simulink model "ILC_controller"  (R2018a)
settings: Solver=VariableStepAuto  StartTime=0.0  StopTime=100  RelTol=1e-3  EnableMultiTasking=on
libraries: simulink x2
settings Model: Creator=HUY  LastModifiedBy=thanhdo
settings OptimizationCC: LifeSpan=inf
settings DebuggingCC: SFUnexpectedBacktrackingDiag=warning  SFNoUnconditionalDefaultTransitionDiag=warning
settings CodeAppCC: StateflowObjectComments=on
settings GRTTargetCC: TargetLangStandard=C89/C90 (ANSI)
settings ConfigComp: CovMetricSettings=dw  CovSaveCumulativeToWorkspaceVar=on  CovSaveSingleToWorkspaceVar=on  CovExternalEMLEnable=off
settings SimscapeCC: SimscapeNormalizeSystem=off

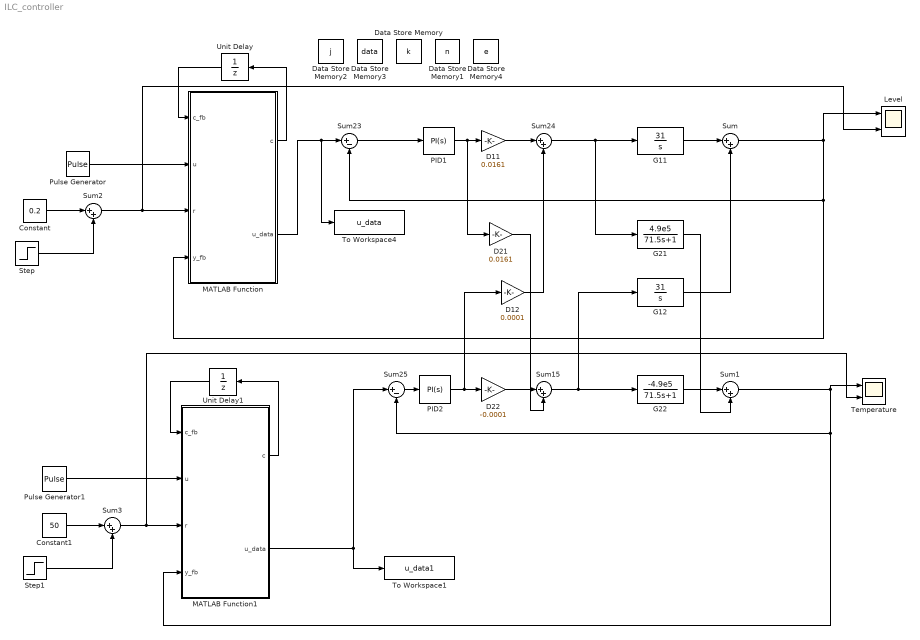
== system ILC_controller ==
  Constant : Constant  Value=0.2
  Constant1 : Constant  Value=50
  D11 : Gain  Gain=0.0161
  D12 : Gain  Gain=0.0001
  D21 : Gain  Gain=0.0161
  D22 : Gain  Gain=-0.0001
  Data Store Memory : DataStoreMemory  DataStoreName=k  ReadBeforeWriteMsg=warning  WriteAfterWriteMsg=warning  WriteAfterReadMsg=warning  ShowAdditionalParam=off  OutDataTypeStr=double
  Data Store Memory1 : DataStoreMemory  DataStoreName=n  ReadBeforeWriteMsg=warning  WriteAfterWriteMsg=warning  WriteAfterReadMsg=warning  ShowAdditionalParam=off  OutDataTypeStr=double
  Data Store Memory2 : DataStoreMemory  DataStoreName=j  ReadBeforeWriteMsg=warning  WriteAfterWriteMsg=warning  WriteAfterReadMsg=warning  ShowAdditionalParam=off  OutDataTypeStr=double
  Data Store Memory3 : DataStoreMemory  DataStoreName=data  ReadBeforeWriteMsg=warning  WriteAfterWriteMsg=warning  WriteAfterReadMsg=warning  ShowAdditionalParam=off  OutDataTypeStr=double  Dimensions=[1 120]
  Data Store Memory4 : DataStoreMemory  DataStoreName=e  ReadBeforeWriteMsg=warning  WriteAfterWriteMsg=warning  WriteAfterReadMsg=warning  ShowAdditionalParam=off  OutDataTypeStr=double  Dimensions=[1 120]
  G11 : TransferFcn  Numerator=[31]  Denominator=[1 0]
  "G12 " : TransferFcn  Numerator=[31]  Denominator=[1 0]
  G21 : TransferFcn  Numerator=[4.9e5]  Denominator=[71.5 1]
  G22 : TransferFcn  Numerator=[-4.9e5]  Denominator=[71.5 1]
  Level : Scope  NumInputPorts=2
  MATLAB Function : MATLAB Function  TreatAsAtomicUnit=on
  MATLAB Function1 : MATLAB Function  TreatAsAtomicUnit=on
  PID1 : simulink/Continuous/PID Controller  Controller=PI  TimeDomain=Continuous-time  SampleTime=-1  IntegratorMethod=Forward Euler  FilterMethod=Forward Euler  Form=Parallel  UseFilter=on  ControllerParametersSource=internal  P=3  I=0.1  D=0  N=100  InitialConditionSource=internal  InitialConditionForIntegrator=0  InitialConditionForFilter=0  ExternalReset=none  LimitOutput=off  UpperSaturationLimit=inf  LowerSaturationLimit=-inf  LinearizeAsGain=on  AntiWindupMode=none  Kb=1  TrackingMode=off  Kt=1  PParamMin=[]  PParamMax=[]  IParamMin=[]  IParamMax=[]  DParamMin=[]  DParamMax=[]  NParamMin=[]  NParamMax=[]  KbParamMin=[]  KbParamMax=[]  KtParamMin=[]  KtParamMax=[]  POutMin=[]  POutMax=[]  IOutMin=[]  IOutMax=[]  DOutMin=[]  DOutMax=[]  NOutMin=[]  NOutMax=[]  KbOutMin=[]  KbOutMax=[]  KtOutMin=[]  KtOutMax=[]  IntegratorOutMin=[]  IntegratorOutMax=[]  FilterOutMin=[]  FilterOutMax=[]  SumOutMin=[]  SumOutMax=[]  SumI1OutMin=[]  SumI1OutMax=[]  SumI2OutMin=[]  SumI2OutMax=[]  SumI3OutMin=[]  SumI3OutMax=[]  SumDOutMin=[]  SumDOutMax=[]  SaturationOutMin=[]  SaturationOutMax=[]  IntegratorContinuousStateAttributes=''  IntegratorStateMustResolveToSignalObject=off  IntegratorRTWStateStorageClass=Auto  FilterContinuousStateAttributes=''  FilterStateMustResolveToSignalObject=off  FilterRTWStateStorageClass=Auto  DifferentiatorICPrevScaledInput=0  DifferentiatorOutMin=[]  DifferentiatorOutMax=[]  FilterDiffOutCoefMin=[]  FilterDiffOutCoefMax=[]  SumDenOutMin=[]  SumDenOutMax=[]  SumNumOutMin=[]  SumNumOutMax=[]  ReciprocalOutMin=[]  ReciprocalOutMax=[]  DivideOutMin=[]  DivideOutMax=[]  TunerSelectOption=Transfer Function Based (PID Tuner App)
  PID2 : simulink/Continuous/PID Controller  Controller=PI  TimeDomain=Continuous-time  SampleTime=-1  IntegratorMethod=Forward Euler  FilterMethod=Forward Euler  Form=Parallel  UseFilter=on  ControllerParametersSource=internal  P=1  I=0.03  D=0  N=100  InitialConditionSource=internal  InitialConditionForIntegrator=0  InitialConditionForFilter=0  ExternalReset=none  LimitOutput=off  UpperSaturationLimit=inf  LowerSaturationLimit=-inf  LinearizeAsGain=on  AntiWindupMode=none  Kb=1  TrackingMode=off  Kt=1  PParamMin=[]  PParamMax=[]  IParamMin=[]  IParamMax=[]  DParamMin=[]  DParamMax=[]  NParamMin=[]  NParamMax=[]  KbParamMin=[]  KbParamMax=[]  KtParamMin=[]  KtParamMax=[]  POutMin=[]  POutMax=[]  IOutMin=[]  IOutMax=[]  DOutMin=[]  DOutMax=[]  NOutMin=[]  NOutMax=[]  KbOutMin=[]  KbOutMax=[]  KtOutMin=[]  KtOutMax=[]  IntegratorOutMin=[]  IntegratorOutMax=[]  FilterOutMin=[]  FilterOutMax=[]  SumOutMin=[]  SumOutMax=[]  SumI1OutMin=[]  SumI1OutMax=[]  SumI2OutMin=[]  SumI2OutMax=[]  SumI3OutMin=[]  SumI3OutMax=[]  SumDOutMin=[]  SumDOutMax=[]  SaturationOutMin=[]  SaturationOutMax=[]  IntegratorContinuousStateAttributes=''  IntegratorStateMustResolveToSignalObject=off  IntegratorRTWStateStorageClass=Auto  FilterContinuousStateAttributes=''  FilterStateMustResolveToSignalObject=off  FilterRTWStateStorageClass=Auto  DifferentiatorICPrevScaledInput=0  DifferentiatorOutMin=[]  DifferentiatorOutMax=[]  FilterDiffOutCoefMin=[]  FilterDiffOutCoefMax=[]  SumDenOutMin=[]  SumDenOutMax=[]  SumNumOutMin=[]  SumNumOutMax=[]  ReciprocalOutMin=[]  ReciprocalOutMax=[]  DivideOutMin=[]  DivideOutMax=[]  TunerSelectOption=Transfer Function Based (PID Tuner App)
  Pulse Generator : DiscretePulseGenerator  PulseType=Time based  Period=0.2  PulseWidth=50  PhaseDelay=0.1
  Pulse Generator1 : DiscretePulseGenerator  PulseType=Time based  Period=0.2  PulseWidth=50  PhaseDelay=0.1
  Step : Step  Time=30  After=0.05  SampleTime=0
  Step1 : Step  Time=50  After=10  SampleTime=0
  Sum{,1..3,15,24} (6 alike) : Sum  Inputs=|++
  Sum23 : Sum  Inputs=|+-
  Sum25 : Sum  Inputs=|+-
  Temperature : Scope  NumInputPorts=2
  To Workspace1 : ToWorkspace  VariableName=u_data1  SampleTime=-1
      settings: Save2DSignal=2-D array (concatenate along first dimension)
  To Workspace4 : ToWorkspace  VariableName=u_data  SampleTime=-1
      settings: Save2DSignal=2-D array (concatenate along first dimension)
  Unit Delay : UnitDelay  InitialCondition=1  SampleTime=-1
  Unit Delay1 : UnitDelay  InitialCondition=1  SampleTime=-1
  wires:
  Sum25/1 -> PID2/1
  D21/1 -> Sum15/2
  D12/1 -> Sum24/2
  Sum23/1 -> PID1/1
  D11/1 -> Sum24/1
  D22/1 -> Sum15/1
  PID1/1 -> D11/1, D21/1
  PID2/1 -> D12/1, D22/1
  Sum1/1 -> Temperature/1, MATLAB Function1/4(y_fb), Sum25/2
  Sum24/1 -> G21/1, G11/1
  G11/1 -> Sum/1
  Sum15/1 -> "G12 "/1, G22/1
  "G12 "/1 -> Sum/2
  G21/1 -> Sum1/2
  G22/1 -> Sum1/1
  Sum/1 -> MATLAB Function/4(y_fb), Sum23/2, Level/1
  MATLAB Function/1(c) -> Unit Delay/1
  Unit Delay/1 -> MATLAB Function/1(c_fb)
  MATLAB Function/2(u_data) -> To Workspace4/1, Sum23/1
  Pulse Generator/1 -> MATLAB Function/2(u)
  MATLAB Function1/1(c) -> Unit Delay1/1
  Unit Delay1/1 -> MATLAB Function1/1(c_fb)
  MATLAB Function1/2(u_data) -> Sum25/1, To Workspace1/1
  Pulse Generator1/1 -> MATLAB Function1/2(u)
  Constant/1 -> Sum2/1
  Step/1 -> Sum2/2
  Sum2/1 -> Level/2, MATLAB Function/3(r)
  Constant1/1 -> Sum3/1
  Step1/1 -> Sum3/2
  Sum3/1 -> Temperature/2, MATLAB Function1/3(r)

== matlab function ILC_controller/MATLAB Function1 ==
  settings: updateMethod=DISCRETE
  data: c_fb input; u input; c output; k data_store_memory; n data_store_memory; j data_store_memory; data data_store_memory; e data_store_memory; r input; y_fb input; u_data output
function [c, u_data] = fcn(c_fb, u, r, y_fb)
c=u;

t=c_fb;y_1=0;
global k n j data e

if t~=u
    k=k+1;
    if k==1
        n=n+1;
    end
end
if rem(k,120)==1 && k>120
    n=n+1; % number of Iterative
end

if n==1 
    j=k; % j index 
elseif n>1
    j=k-(n-1)*120;
end


if n==1
    if j==1
        e(j)=r-y_1;% error e=r-y_fb
    else
        e(j)=r-y_fb;% error e=r-y_fb
    end
    data(j)=r+0.1*e(j); %correction formula u(i)=u(i)+k*r with iterative n=1 replace u(i)=> r
elseif n>=2 
    e(j)=r-y_fb;
    data(j)=data(j)+0.1*e(j); 
end

u_data=data(j); % send u_dk to plant

== matlab function ILC_controller/MATLAB Function ==
  settings: updateMethod=DISCRETE
  data: c_fb input; u input; c output; k data_store_memory; n data_store_memory; j data_store_memory; data data_store_memory; e data_store_memory; r input; y_fb input; u_data output
function [c, u_data] = fcn(c_fb, u, r, y_fb)
c=u;

t=c_fb;y_1=0;
global k n j data e

if t~=u
    k=k+1;
    if k==1
        n=n+1;
    end
end
if rem(k,120)==1 && k>120
    n=n+1; % number of Iterative
end

if n==1 
    j=k; % j index 
elseif n>1
    j=k-(n-1)*120;
end


if n==1
    if j==1
        e(j)=r-y_1;% error e=r-y_fb
    else
        e(j)=r-y_fb;% error e=r-y_fb
    end
    data(j)=r+0.05*e(j); %correction formula u(i)=u(i)+k*r with iterative n=1 replace u(i)=> r
elseif n>=2 
    e(j)=r-y_fb;
    data(j)=data(j)+0.05*e(j); 
end

u_data=data(j); % send u_dk to plant
